simulink library "carnot"  (R2018b)
settings: Solver=VariableStepAuto  StartTime=0.0  StopTime=10.0  RelTol=1e-3
undefined symbols (not defined in the file or in its folder): A, A_earth, acol, Acol, ActPower1, ActPower2, ActPower3, Ad, Ad0, Ar, Au, Au0, Azimuth_Angle, B, Bd, Bd0, Br, Bu, Bu0, C, c1, c2, c3, c33, c4, c5, c6, CarnotCallbacks_Density, CarnotCallbacks_Enthalpy, CarnotCallbacks_Enthalpy2Temperature, CarnotCallbacks_Entropy, CarnotCallbacks_Evaporation_Enthalpy, CarnotCallbacks_GlobalMessageLevel, CarnotCallbacks_Grashof, CarnotCallbacks_Heat_Capacity, CarnotCallbacks_Kinematic_Viscosity, CarnotCallbacks_PMV_PPD, CarnotCallbacks_Prandtl, CarnotCallbacks_Saturation_Property, CarnotCallbacks_Saturation_Temperature, CarnotCallbacks_Saturation_Value_Water, CarnotCallbacks_Specific_Volume, CarnotCallbacks_Thermal_Conductivity, CarnotCallbacks_Vapour_Content, CarnotCallbacks_Vapour_Pressure, Cd, Cdl, Cr, Cu, Davies, Dd, DE_TRY2010_04_averageYear, delta_grd, density, DiameterLastPiece, dl, DPConstant, DPLinear, DPQuadratic, Dr ... (+59)
libraries: $bdroot x429, simulink x36, simulink_extras x12
(part 14 of 22)

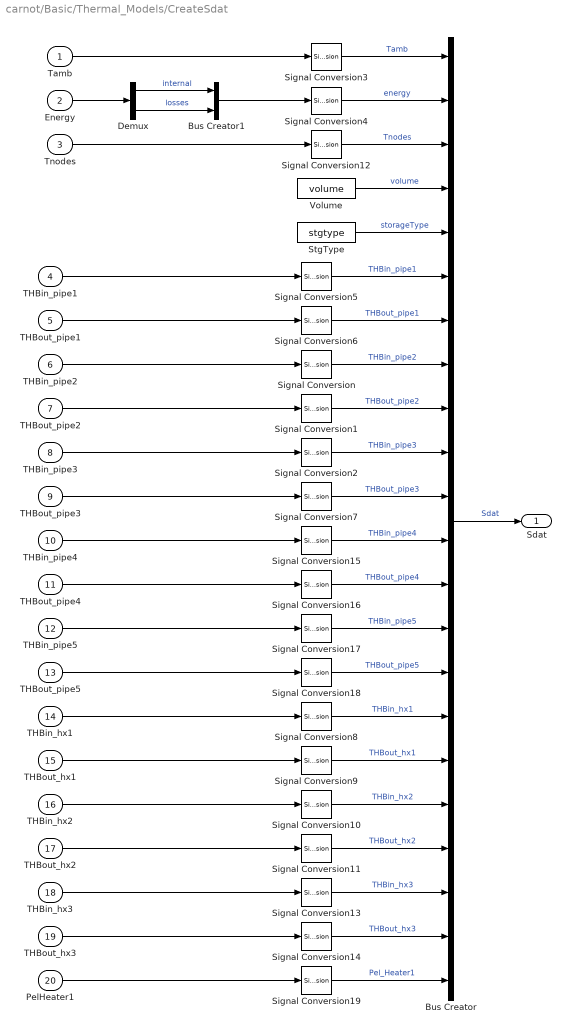
== system carnot/Basic/Thermal_Models/CreateSdat ==
  Tamb : Inport
  Energy : Inport  Port=2
  Tnodes : Inport  Port=3
  THBin_pipe1 : Inport  Port=4
  THBout_pipe1 : Inport  Port=5
  THBin_pipe2 : Inport  Port=6
  THBout_pipe2 : Inport  Port=7
  THBin_pipe3 : Inport  Port=8
  THBout_pipe3 : Inport  Port=9
  THBin_pipe4 : Inport  Port=10
  THBout_pipe4 : Inport  Port=11
  THBin_pipe5 : Inport  Port=12
  THBout_pipe5 : Inport  Port=13
  THBin_hx1 : Inport  Port=14
  THBout_hx1 : Inport  Port=15
  THBin_hx2 : Inport  Port=16
  THBout_hx2 : Inport  Port=17
  THBin_hx3 : Inport  Port=18
  THBout_hx3 : Inport  Port=19
  PelHeater1 : Inport  Port=20
  Bus Creator : BusCreator  Inputs=22
  Bus Creator1 : BusCreator  Inputs=2
  Demux : Demux  Outputs=2
  Signal Conversion{,1..19} (20 alike) : SignalConversion  OverrideOpt=off
  StgType : Constant  Value=stgtype
  Volume : Constant  Value=volume
  Sdat : Outport
  wires:
  Volume/1 -> Bus Creator/4  "volume"
  Bus Creator1/1 -> Signal Conversion4/1
  Energy/1 -> Demux/1
  Demux/1 -> Bus Creator1/1  "internal"
  Demux/2 -> Bus Creator1/2  "losses"
  Signal Conversion3/1 -> Bus Creator/1  "Tamb"
  THBin_pipe2/1 -> Signal Conversion/1
  Signal Conversion5/1 -> Bus Creator/6  "THBin_pipe1"
  Signal Conversion7/1 -> Bus Creator/11  "THBout_pipe3"
  THBout_pipe3/1 -> Signal Conversion7/1
  Signal Conversion10/1 -> Bus Creator/18  "THBin_hx2"
  Tnodes/1 -> Signal Conversion12/1
  THBin_pipe3/1 -> Signal Conversion2/1
  Tamb/1 -> Signal Conversion3/1
  Signal Conversion8/1 -> Bus Creator/16  "THBin_hx1"
  Signal Conversion4/1 -> Bus Creator/2  "energy"
  Signal Conversion9/1 -> Bus Creator/17  "THBout_hx1"
  THBout_pipe2/1 -> Signal Conversion1/1
  Signal Conversion6/1 -> Bus Creator/7  "THBout_pipe1"
  Signal Conversion12/1 -> Bus Creator/3  "Tnodes"
  THBin_hx1/1 -> Signal Conversion8/1
  THBout_hx1/1 -> Signal Conversion9/1
  THBin_hx2/1 -> Signal Conversion10/1
  Bus Creator/1 -> Sdat/1  "Sdat"
  THBin_pipe1/1 -> Signal Conversion5/1
  THBout_hx2/1 -> Signal Conversion11/1
  THBout_pipe1/1 -> Signal Conversion6/1
  Signal Conversion1/1 -> Bus Creator/9  "THBout_pipe2"
  Signal Conversion/1 -> Bus Creator/8  "THBin_pipe2"
  Signal Conversion2/1 -> Bus Creator/10  "THBin_pipe3"
  Signal Conversion11/1 -> Bus Creator/19  "THBout_hx2"
  Signal Conversion13/1 -> Bus Creator/20  "THBin_hx3"
  THBin_hx3/1 -> Signal Conversion13/1
  THBout_hx3/1 -> Signal Conversion14/1
  Signal Conversion14/1 -> Bus Creator/21  "THBout_hx3"
  StgType/1 -> Bus Creator/5  "storageType"
  Signal Conversion15/1 -> Bus Creator/12  "THBin_pipe4"
  THBin_pipe4/1 -> Signal Conversion15/1
  THBout_pipe4/1 -> Signal Conversion16/1
  Signal Conversion16/1 -> Bus Creator/13  "THBout_pipe4"
  Signal Conversion18/1 -> Bus Creator/15  "THBout_pipe5"
  THBout_pipe5/1 -> Signal Conversion18/1
  THBin_pipe5/1 -> Signal Conversion17/1
  Signal Conversion17/1 -> Bus Creator/14  "THBin_pipe5"
  PelHeater1/1 -> Signal Conversion19/1
  Signal Conversion19/1 -> Bus Creator/22  "Pel_Heater1"

== system carnot/Basic/Thermal_Models/Floor_in ==
  "[AIV]floor" : Inport
  power per node : Inport  Port=2
  "[AIV]ceiling" : Inport  Port=3
  Qdot_sol : Inport  Port=4
  Mux : Mux  Inputs=3
  Wall_basic : $bdroot/Basic/Thermal_Models/Wall_basic  tau=tau  t0=t0  d=d  dactive=dactive  cond=cond  cwall=cwall  rho=rho
  alfa_ceiling : $bdroot/Basic/Heat_Transfer/alfa_ceiling  active=active  emission_c=emission_c  wallsurface=wallsurface
  alfa_floor : $bdroot/Basic/Heat_Transfer/alfa_floor  active=active  emission_f=emission_f  wallsurface=wallsurface
  per surface : Gain  Gain=1/wallsurface  SaturateOnIntegerOverflow=on  OutDataTypeStr=Inherit: Same as input  ParamDataTypeStr=Inherit: Same as input
  "[S]floor" : Outport
  T(P) : Outport  Port=2
  "[S]ceiling" : Outport  Port=3
  Tn : Outport  Port=4
  wires:
  Wall_basic/2 -> Mux/2, T(P)/1
  "[AIV]ceiling"/1 -> alfa_ceiling/2
  alfa_ceiling/2 -> "[S]ceiling"/1
  alfa_floor/2 -> "[S]floor"/1
  "[AIV]floor"/1 -> alfa_floor/2
  Wall_basic/3 -> Mux/3, alfa_ceiling/1
  Wall_basic/1 -> Mux/1, alfa_floor/1
  alfa_floor/1 -> Wall_basic/1
  alfa_ceiling/1 -> Wall_basic/3
  Qdot_sol/1 -> alfa_floor/3
  power per node/1 -> per surface/1
  per surface/1 -> Wall_basic/2
  Mux/1 -> Tn/1

== system carnot/Basic/Thermal_Models/HeatPump_basic ==
  THBin_source : Inport
  THBin_load : Inport  Port=2
  Tamb : Inport  Port=3
  Ctrl : Inport  Port=4
  Bus Assignment : BusAssignment  AssignedSignals=Temperature
  Bus Assignment1 : BusAssignment  AssignedSignals=Temperature
  Bus Creator : BusCreator  Inputs=7
  Bus Selector : BusSelector  OutputSignals=Temperature,MassFlow,Pressure,FluidType,FluidMix
  Bus Selector1 : BusSelector  OutputSignals=Temperature,MassFlow,Pressure,FluidType,FluidMix
  P_el calculus : Subsystem
  Product : DotProduct  InputSameDT=on  OutDataTypeStr=Inherit: Inherit via internal rule
  Product1 : DotProduct  InputSameDT=on  OutDataTypeStr=Inherit: Inherit via internal rule
  Product3 : DotProduct  InputSameDT=on  OutDataTypeStr=Inherit: Inherit via internal rule
  Sum1 : Sum  Inputs=+-  SaturateOnIntegerOverflow=on  InputSameDT=on  OutDataTypeStr=Inherit: Same as first input
  Sum2 : Sum  Inputs=+-  SaturateOnIntegerOverflow=on  InputSameDT=on  OutDataTypeStr=Inherit: Same as first input
  model cold side : Subsystem
  model hot side : Subsystem
  THBsource : Outport
  THBload : Outport  Port=2
  HPdat : Outport  Port=3
  wires:
  Product/1 -> Bus Creator/6  "Qdot_hot"
  Product3/1 -> Bus Creator/3  "Qdot_cold"
  model cold side/2(mdot*cp) -> Product3/2
  Sum1/1 -> Product3/1
  Bus Selector1/2 -> model cold side/2(mdot_cold)  "<MassFlow>"
  Ctrl/1 -> model hot side/8(command), Product1/1, model cold side/8(command)
  model hot side/2(Thot_out) -> Sum2/1, P_el calculus/1(Thot_out), model cold side/6(Thot), Bus Assignment/2
  Product1/1 -> Bus Creator/7  "Pelec"
  P_el calculus/1(P_el) -> Product1/2
  Bus Selector/3 -> model hot side/4(p_hot)  "<Pressure>"
  model cold side/1(Tcold_out) -> Bus Assignment1/2, Sum1/2
  Bus Selector1/1 -> model cold side/1(Tcold), Sum1/1, model hot side/1(Tcold), P_el calculus/2(Tcold_in)  "<Temperature>"
  Sum2/1 -> Product/2
  model hot side/1(mdot*cp) -> Product/1
  Bus Selector/2 -> model hot side/3(mdot_hot)  "<MassFlow>"
  Bus Selector/1 -> model hot side/2(Thot), Sum2/2  "<Temperature>"
  Bus Selector/5 -> model hot side/6(mix_hot)  "<FluidMix>"
  Bus Selector/4 -> model hot side/5(fluid_hot)  "<FluidType>"
  Bus Selector1/3 -> model cold side/3(p_cold)  "<Pressure>"
  Bus Selector1/4 -> model cold side/4(fluid_cold)  "<FluidType>"
  Bus Selector1/5 -> model cold side/5(mix_cold)  "<FluidMix>"
  THBin_load/1 -> Bus Selector/1, Bus Assignment/1, Bus Creator/4  "THBin_hot"
  Tamb/1 -> model cold side/7(Tamb), model hot side/7(Tamb)
  Bus Assignment/1 -> THBload/1, Bus Creator/5  "THBout_hot"
  THBin_source/1 -> Bus Selector1/1, Bus Assignment1/1, Bus Creator/1  "THBin_cold"
  Bus Assignment1/1 -> THBsource/1, Bus Creator/2  "THBout_cold"
  Bus Creator/1 -> HPdat/1

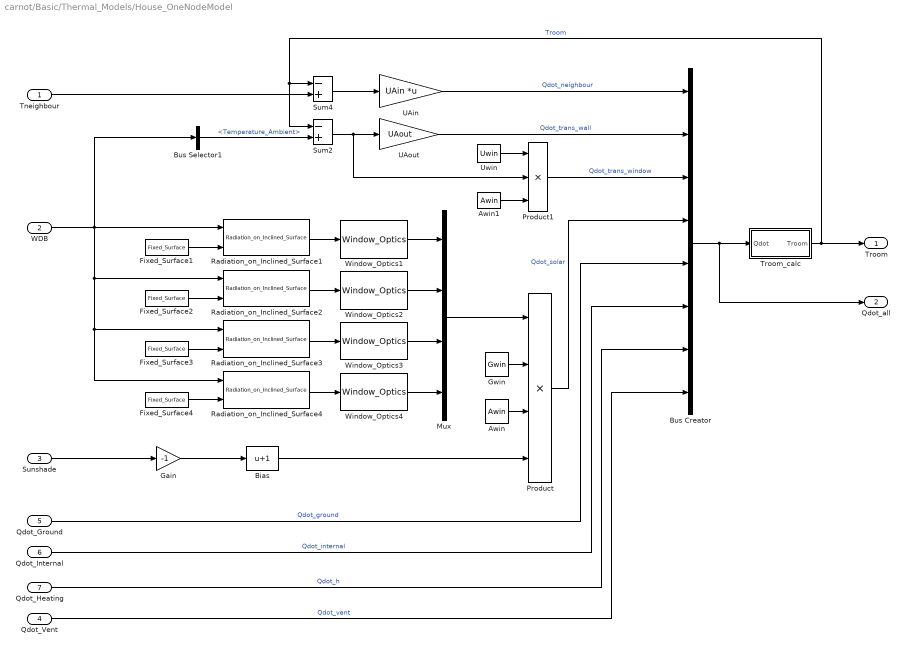
== system carnot/Basic/Thermal_Models/House_OneNodeModel ==
  Tneighbour : Inport
  WDB : Inport  Port=2
  Sunshade : Inport  Port=3
  Qdot_Vent : Inport  Port=4
  Qdot_Ground : Inport  Port=5
  Qdot_Internal : Inport  Port=6
  Qdot_Heating : Inport  Port=7
  Awin : Constant  Value=Awin
  Awin1 : Constant  Value=Awin
  Bias : Bias  Bias=1
  Bus Creator : BusCreator  Inputs=8
  Bus Selector1 : BusSelector  OutputSignals=Temperature_Ambient
  Fixed_Surface1 : $bdroot/Weather/Fixed_Surface  colangle=90  colazi=AziWin(1)  colrot=0
  Fixed_Surface2 : $bdroot/Weather/Fixed_Surface  colangle=90  colazi=AziWin(2)  colrot=0
  Fixed_Surface3 : $bdroot/Weather/Fixed_Surface  colangle=90  colazi=AziWin(3)  colrot=0
  Fixed_Surface4 : $bdroot/Weather/Fixed_Surface  colangle=90  colazi=AziWin(4)  colrot=0
  Gain : Gain  Gain=-1
  Gwin : Constant  Value=Gwin
  Mux : Mux
  Product : Product  Inputs=4
  Product1 : Product  Inputs=3
  Radiation_on_Inclined_Surface{1..4} (4 alike) : $bdroot/Weather/Radiation_on_Inclined_Surface  sky=Perez 1990  reflect=0.2
  Sum2 : Sum  Inputs=-+  SaturateOnIntegerOverflow=on  InputSameDT=on  OutDataTypeStr=Inherit: Same as first input
  Sum4 : Sum  Inputs=-+  SaturateOnIntegerOverflow=on  InputSameDT=on  OutDataTypeStr=Inherit: Same as first input
  Troom_calc : Subsystem  mask(Calculate room temperature){A=A, capa=capa, tini=tini, dtroom=dtroom}
      mask prompts: A "Heated surface of the house in m²"; capa "Thermal capactiy per surface in J/m²/K"; tini "Initial temperature in °C"; dtroom "Max. change of room temperature in K"
      mask help:
      | One node thermal model based on energy balance.
      | The room temperature can be limited by "Max. change of room temperature" . The temperature is limited by this parameter, the result of the energy balance (Qdot_all) is the required power to maintain the limit.
      mask TypeOptions A: A/Value
      mask TypeOptions capa: capa/Value
      mask TypeOptions tini: Tini/Value | add_Tini/Bias
  UAin : Gain  Gain=UAin  Multiplication=Matrix(K*u)  SaturateOnIntegerOverflow=on  OutDataTypeStr=Inherit: Same as input  ParamDataTypeStr=Inherit: Same as input
  UAout : Gain  Gain=UAout  SaturateOnIntegerOverflow=on  OutDataTypeStr=Inherit: Same as input  ParamDataTypeStr=Inherit: Same as input
  Uwin : Constant  Value=Uwin
  Window_Optics{1..4} (4 alike) : $bdroot/Basic/Thermal_Models/Window_Optics  BreakpointsForDimension1=[-10 0 50 70 80 90]  Table="[1.0 1.0  0.95  0.7  0.0  0.0]"  Gain=0.8
  Troom : Outport
  Qdot_all : Outport  Port=2
  wires:
  Bias/1 -> Product/4
  Gain/1 -> Bias/1
  Uwin/1 -> Product1/1
  Awin1/1 -> Product1/3
  Awin/1 -> Product/3
  Gwin/1 -> Product/2
  Tneighbour/1 -> Sum4/2
  Qdot_Vent/1 -> Bus Creator/8  "Qdot_vent"
  Sunshade/1 -> Gain/1
  Mux/1 -> Product/1
  Qdot_Heating/1 -> Bus Creator/7  "Qdot_h"
  Window_Optics4/1 -> Mux/4
  Window_Optics3/1 -> Mux/3
  Window_Optics2/1 -> Mux/2
  Window_Optics1/1 -> Mux/1
  Product/1 -> Bus Creator/4  "Qdot_solar"
  Sum2/1 -> UAout/1, Product1/2
  UAout/1 -> Bus Creator/2  "Qdot_trans_wall"
  Bus Selector1/1 -> Sum2/2  "<Temperature_Ambient>"
  WDB/1 -> Bus Selector1/1, Radiation_on_Inclined_Surface4/1, Radiation_on_Inclined_Surface3/1, Radiation_on_Inclined_Surface2/1, Radiation_on_Inclined_Surface1/1
  Bus Creator/1 -> Qdot_all/1, Troom_calc/1(Qdot)
  Qdot_Ground/1 -> Bus Creator/5  "Qdot_ground"
  Sum4/1 -> UAin/1
  UAin/1 -> Bus Creator/1  "Qdot_neighbour"
  Fixed_Surface1/1 -> Radiation_on_Inclined_Surface1/2
  Radiation_on_Inclined_Surface1/1 -> Window_Optics1/1
  Fixed_Surface2/1 -> Radiation_on_Inclined_Surface2/2
  Radiation_on_Inclined_Surface2/1 -> Window_Optics2/1
  Fixed_Surface3/1 -> Radiation_on_Inclined_Surface3/2
  Radiation_on_Inclined_Surface3/1 -> Window_Optics3/1
  Fixed_Surface4/1 -> Radiation_on_Inclined_Surface4/2
  Radiation_on_Inclined_Surface4/1 -> Window_Optics4/1
  Troom_calc/1(Troom) -> Troom/1, Sum4/1, Sum2/1  "Troom"
  Product1/1 -> Bus Creator/3  "Qdot_trans_window"
  Qdot_Internal/1 -> Bus Creator/6  "Qdot_internal"

== system carnot/Basic/Thermal_Models/Pipe_basic ==
  Tamb : Inport
  THBin : Inport  Port=2
  Bus Assignment : BusAssignment  AssignedSignals=Temperature
  Bus Selector : BusSelector  OutputSignals=Temperature,MassFlow,Pressure,FluidType,FluidMix
  S-Function : S-Function  FunctionName=pipe_Tnodes  Parameters="vnode, lnode,  unode,  cond,  cnode,  t0, nodes"  SFunctionDeploymentMode=off  EnableBusSupport=off
  Tnodes : Outport
  THB : Outport  Port=2
  wires:
  THBin/1 -> Bus Assignment/1, Bus Selector/1
  S-Function/1 -> Bus Assignment/2
  Tamb/1 -> S-Function/1
  Bus Selector/1 -> S-Function/2  "<Temperature>"
  Bus Selector/2 -> S-Function/3  "<MassFlow>"
  Bus Selector/3 -> S-Function/4  "<Pressure>"
  Bus Selector/4 -> S-Function/5  "<FluidType>"
  Bus Selector/5 -> S-Function/6  "<FluidMix>"
  S-Function/2 -> Tnodes/1
  Bus Assignment/1 -> THB/1

== system carnot/Basic/Thermal_Models/Radiator_basic ==
  note: One node model with upwind scheme. Power balance is:
      | m*cp*dTnode/dt = -qdot + mdot*cp*(Tin - Tnode)
      |
      | EN 442:
      | qdot = qdot_nominal * ((Tnode-Troom)/(Tdiff_nominal)^expo
      | nominal temperature difference = 50K with flowline 75°C, return 65°C and room 20°C
      | in EN, the Tnode is mean temperature Tm = 0.5*(Tin+Tout)
      |
      | Here Tout = Tnode in difference to EN442
      | A correction of expo and nominal power is done in the mask.
  THB_in : Inport
  Troom : Inport  Port=2
  Abs : Abs  SaturateOnIntegerOverflow=on
  Bus Selector : BusSelector  OutputSignals=Temperature,MassFlow
  Gain : Gain  Gain=1/dtnom  SaturateOnIntegerOverflow=on  OutDataTypeStr=Inherit: Same as input  ParamDataTypeStr=Inherit: Same as input
  Gain1 : Gain  Gain=pnom  SaturateOnIntegerOverflow=on  OutDataTypeStr=Inherit: Same as input  ParamDataTypeStr=Inherit: Same as input
  Heat_Capacity : $bdroot/Basic/Material_Properties/Heat_Capacity  VariantControl=CarlibClassic  INPUTARGUMENTS=THB  DEBUGLEVEL=DEBUGLEVEL  MAXTOTALWARNINGS=inf  MAXCONSECUTIVEWARNINGS=inf  WRITETOFILE=0  FILENAME='errors.txt'
  Math Function : Math  Operator=pow  SaturateOnIntegerOverflow=on
  Product : Product  Inputs=3  SaturateOnIntegerOverflow=on  InputSameDT=on  OutDataTypeStr=Inherit: Same as first input
  Product1 : Product  SaturateOnIntegerOverflow=on  InputSameDT=on  OutDataTypeStr=Inherit: Same as first input
  Sign : Signum
  Sum : Sum  Inputs=-+  SaturateOnIntegerOverflow=on  InputSameDT=on  OutDataTypeStr=Inherit: Same as first input
  Sum1 : Sum  Inputs=-+  SaturateOnIntegerOverflow=on  InputSameDT=on  OutDataTypeStr=Inherit: Same as first input
  Sum3 : Sum  Inputs=-+  SaturateOnIntegerOverflow=on  InputSameDT=on  OutDataTypeStr=Inherit: Same as first input
  THB_set_T : $bdroot/Source/Simple/THB_set_T
  Transfer Fcn (with initial states) : simulink_extras/Additional Linear/Transfer Fcn (with initial states)  N=[1]  D="[mcap  0]"  X0=tini*mcap
  const : Constant  Value=expo
  THB : Outport
  Qdot2room : Outport  Port=2
  wires:
  Troom/1 -> Sum3/1
  Bus Selector/1 -> Sum/2  "<Temperature>"
  Sign/1 -> Product1/2
  Sum3/1 -> Sign/1, Gain/1
  Gain1/1 -> Product1/1
  Abs/1 -> Math Function/1
  Gain/1 -> Abs/1
  Math Function/1 -> Gain1/1
  const/1 -> Math Function/2
  Product1/1 -> Qdot2room/1, Sum1/1
  Sum/1 -> Product/1
  Bus Selector/2 -> Product/2  "<MassFlow>"
  Heat_Capacity/1 -> Product/3
  Product/1 -> Sum1/2
  Sum1/1 -> Transfer Fcn (with initial states)/1
  Transfer Fcn (with initial states)/1 -> Sum3/2, Sum/1, THB_set_T/2
  THB_set_T/1 -> THB/1
  THB_in/1 -> Bus Selector/1, Heat_Capacity/1, THB_set_T/1

== system carnot/Basic/Thermal_Models/Roof ==
  WDB : Inport
  power per node : Inport  Port=2
  "[AIV]" : Inport  Port=3
  Mux : Mux  Inputs=3
  Wall_basic : $bdroot/Basic/Thermal_Models/Wall_basic  tau=tau  t0=t0  d=d  dactive=dactive  cond=cond  cwall=cwall  rho=rho
  alfa_ceiling : $bdroot/Basic/Heat_Transfer/alfa_ceiling  active=active  emission_c=emission_c  wallsurface=wallsurface
  alfa_wall_out : $bdroot/Basic/Heat_Transfer/alfa_wall_out  pos=pos  absorption_out=absorption_out  emission_out=emission_out  wallsurface=wallsurface
  per surface : Gain  Gain=1/wallsurface  SaturateOnIntegerOverflow=on  OutDataTypeStr=Inherit: Same as input  ParamDataTypeStr=Inherit: Same as input
  "[S]" : Outport
  Tn : Outport  Port=2
  wires:
  per surface/1 -> Wall_basic/2
  power per node/1 -> per surface/1
  alfa_ceiling/2 -> "[S]"/1
  "[AIV]"/1 -> alfa_ceiling/2
  alfa_ceiling/1 -> Wall_basic/3
  Wall_basic/2 -> Mux/2
  Wall_basic/3 -> Mux/3, alfa_ceiling/1
  Wall_basic/1 -> Mux/1, alfa_wall_out/2
  WDB/1 -> alfa_wall_out/1
  alfa_wall_out/1 -> Wall_basic/1
  Mux/1 -> Tn/1

== system carnot/Basic/Thermal_Models/Room_Node ==
  note: NODE of a ZONE ( heat flow, temperature, ventilation / infiltration and energy consumption)
  note: r: radiative
      | c: convective
  sum([S]) : Inport
  1/s to 1/h : Gain  Gain=3600  SaturateOnIntegerOverflow=on  OutDataTypeStr=Inherit: Same as input  ParamDataTypeStr=Inherit: Same as input
  Demux2 : Demux  Outputs=13
  Mux2 : Mux  Inputs=6
  Mux3 : Mux  Inputs=9
  Sensitive room temperature : Subsystem  mask(SENSITIVE TEMPERATURE){share_c=47}
      mask prompts: share_c "SHARE of convective sensitivity, [0,100%]:"
      mask help:
      | This block merges the convective and radiative zone node temperature to the SENSITIVE ZONE TEMPERATURE (weighted arithmetic average of both components).
      |
      | [T] = [Tc; Tr]:  temperature vector of node, °C
      | Ts:              sensitive zone temperature, °C
      mask init: same as carnot/Outputs/Sensitive_Room_Temperature
  Terminator : Terminator
  convective_node : Subsystem
  m^3 : Constant  Value=zoneairvolume
  radiative_node : Subsystem
  "[AIV]" : Outport
  "[S]" : Outport  Port=2
  Qdot_sol : Outport  Port=3
  Vair : Outport  Port=4
  wires:
  Sensitive room temperature/1(Ts) -> Mux3/1  "Ts"
  Mux3/1 -> "[AIV]"/1
  Demux2/13 -> convective_node/6(Vdot_in2out)  "Vdot_in2out"
  Demux2/12 -> convective_node/5(Vdot_out2in)  "Vdot_out2in"
  Demux2/11 -> convective_node/4(D_mdot_CO2)  "delta_mdot_CO2"
  Demux2/10 -> convective_node/3(D_mdot_H2O)  "delta_mdot_H2O"
  Demux2/9 -> convective_node/2(D_mdot_air)  "delta_mdot_air"
  radiative_node/1(Tr) -> Mux3/3, Sensitive room temperature/1(Tr)  "Tr"
  convective_node/1(Tc) -> Mux3/2, Sensitive room temperature/2(Tc)  "Tc"
  convective_node/7(nair_out) -> 1/s to 1/h/1
  convective_node/4(rho) -> Mux3/6  "rho"
  convective_node/5(cp) -> Mux3/7  "cp"
  convective_node/6(p) -> Mux3/8  "p"
  convective_node/3(x_CO2) -> Mux3/5  "x_CO2"
  convective_node/2(x_H2O) -> Mux3/4  "x_H2O"
  1/s to 1/h/1 -> Mux3/9  "nair_out"
  Demux2/1 -> Qdot_sol/1, Mux2/1  "Qdot_sol"
  Demux2/2 -> Mux2/2  "Qdot_equip"
  Demux2/3 -> Mux2/3  "Qdot_light"
  Demux2/4 -> Mux2/4  "Qdot_pers"
  Demux2/5 -> Mux2/5  "Qdot_heat"
  Demux2/6 -> Mux2/6  "Qdot_air"
  Demux2/7 -> convective_node/1(Qdotc)  "Qdotc"
  Demux2/8 -> radiative_node/1(Qdotr)  "Qdotr"
  sum([S])/1 -> Demux2/1, "[S]"/1
  Mux2/1 -> Terminator/1  "[Qdot]"
  m^3/1 -> Vair/1

== system carnot/Basic/Thermal_Models/Solar_Collector_basic ==
  solar : Inport
  THB : Inport  Port=2
  Bus Selector1 : BusSelector  OutputSignals=Temperature,MassFlow
  Bus Selector2 : BusSelector  OutputSignals=Pressure,FluidType,FluidMix  OutputAsBus=on
  S-Function : S-Function  FunctionName=solarcollector12975  Parameters=acol, c1, c2, c3, c4, c5, c6, tini  SFunctionDeploymentMode=off  EnableBusSupport=off
  Tout : Outport
  Tmean : Outport  Port=2
  Qdot : Outport  Port=3
  wires:
  Bus Selector1/2 -> S-Function/3  "<MassFlow>"
  Bus Selector1/1 -> S-Function/2  "<Temperature>"
  Bus Selector2/1 -> S-Function/4
  THB/1 -> Bus Selector1/1, Bus Selector2/1
  solar/1 -> S-Function/1
  S-Function/1 -> Tout/1  "Tout"
  S-Function/2 -> Tmean/1  "Tmean"
  S-Function/3 -> Qdot/1  "power"

== system carnot/Basic/Thermal_Models/T_Ground_Undisturbed ==
  note: u(1) - u(2)*exp(-u(3)/u(4))*cos(2*pi*(u(5)-u(6)*3600)/(365*24*3600) - u(3)/u(4)) + 0.03*u(3)
  -1/delta_grd : Gain  Gain=-1/delta_grd
  Math Function : Math  SaturateOnIntegerOverflow=on
  Product : Product  RndMeth=Zero
  Sine Wave : Sin  Amplitude=deltathetae  Frequency=2*pi/(365*24*3600)  Phase=pi/2 - 2*pi*tshift/(365*24) - z/delta_grd  SampleTime=0
  Sum : Sum  Inputs=+-+
  Tmeanoutside1 : Constant  Value=Tmeanoutside
  gain : Gain  Gain=0.03
  height vector : Constant  Value=z
  Tearth : Outport
  wires:
  Tmeanoutside1/1 -> Sum/1
  Sum/1 -> Tearth/1
  Product/1 -> Sum/2
  Sine Wave/1 -> Product/2
  Math Function/1 -> Product/1
  -1/delta_grd/1 -> Math Function/1
  height vector/1 -> -1/delta_grd/1, gain/1
  gain/1 -> Sum/3

== system carnot/Basic/Thermal_Models/ThermalNodeTHB ==
  THB : Inport
  Bus Selector : BusSelector  OutputSignals=Temperature,MassFlow
  Const : Constant  Value=0
  Heat_Capacity : $bdroot/Basic/Material_Properties/Heat_Capacity  VariantControl=CarlibClassic  INPUTARGUMENTS=THB  DEBUGLEVEL=DEBUGLEVEL  MAXTOTALWARNINGS=inf  MAXCONSECUTIVEWARNINGS=inf  WRITETOFILE=0  FILENAME='errors.txt'
  Tamb : Constant  Value=Tini
  Thermal_Node : $bdroot/Basic/Thermal_Models/Thermal_Node  UA=UA  mcp=mcp
  T : Outport  InitialOutput=20
  wires:
  Tamb/1 -> Thermal_Node/1
  Heat_Capacity/1 -> Thermal_Node/5
  THB/1 -> Heat_Capacity/1, Bus Selector/1
  Bus Selector/2 -> Thermal_Node/3  "<MassFlow>"
  Bus Selector/1 -> Thermal_Node/2  "<Temperature>"
  Thermal_Node/1 -> T/1
  Const/1 -> Thermal_Node/4

== system carnot/Basic/Thermal_Models/Thermal_Node ==
  Tamb : Inport
  Tin : Inport  Port=2
  mdot : Inport  Port=3
  Qdot : Inport  Port=4
  cp : Inport  Port=5
  Divide : Product  Inputs=*/
  Integrator : Integrator  InitialConditionSource=external  InitialCondition=40
  Losses : Gain  Gain=UA  SaturateOnIntegerOverflow=on  OutDataTypeStr=Inherit: Same as input  ParamDataTypeStr=Inherit: Same as input
  Mux : Mux  Inputs=3
  Product1 : Product  Inputs=3  SaturateOnIntegerOverflow=on  InputSameDT=on  OutDataTypeStr=Inherit: Same as first input
  Sum1 : Sum  Inputs=-+  SaturateOnIntegerOverflow=on  InputSameDT=on  OutDataTypeStr=Inherit: Same as first input
  Sum3 : Sum  Inputs=-+  SaturateOnIntegerOverflow=on  InputSameDT=on  OutDataTypeStr=Inherit: Same as first input
  Sum4 : Sum  Inputs=1  SaturateOnIntegerOverflow=on  InputSameDT=on  OutDataTypeStr=Inherit: Same as first input
  nodeCapacity : Constant  Value=mcp
  Tout : Outport  InitialOutput=40
  wires:
  Sum4/1 -> Divide/1
  nodeCapacity/1 -> Divide/2
  mdot/1 -> Product1/2
  Tin/1 -> Sum1/2
  Integrator/1 -> Tout/1, Sum1/1, Sum3/1  "Tout"
  Product1/1 -> Mux/2
  Mux/1 -> Sum4/1
  Tamb/1 -> Sum3/2, Integrator/2
  Losses/1 -> Mux/1
  Sum3/1 -> Losses/1
  cp/1 -> Product1/3
  Divide/1 -> Integrator/1
  Sum1/1 -> Product1/1
  Qdot/1 -> Mux/3

== system carnot/Basic/Thermal_Models/Wall_basic ==
  qdot_in : Inport
  QdotActive : Inport  Port=2
  qdot_out : Inport  Port=3
  S-Function : S-Function  FunctionName=layerwall  Parameters=tau, t0, d, cond, cwall, rho, dactive  SFunctionDeploymentMode=off  EnableBusSupport=off
  Tin : Outport
  Tactive : Outport  Port=2
  Tout : Outport  Port=3
  wires:
  qdot_in/1 -> S-Function/1
  S-Function/1 -> Tin/1
  QdotActive/1 -> S-Function/2
  S-Function/2 -> Tactive/1  "T(active)"
  qdot_out/1 -> S-Function/3
  S-Function/3 -> Tout/1

== system carnot/Basic/Thermal_Models/Wall_in ==
  "[AIV]" : Inport
  power per node : Inport  Port=2
  "[AIV]n" : Inport  Port=3
  Mux : Mux  Inputs=3
  Wall_basic : $bdroot/Basic/Thermal_Models/Wall_basic  tau=tau  t0=t0  d=d  dactive=dactive  cond=cond  cwall=cwall  rho=rho
  alfa_wall_in : $bdroot/Basic/Heat_Transfer/alfa_wall_in  active=active  emission_in=emission_in  wallsurface=wallsurface
  alfa_wall_in1 : $bdroot/Basic/Heat_Transfer/alfa_wall_in  active=active  emission_in=emission_in  wallsurface=wallsurface
  per surface : Gain  Gain=1/wallsurface  SaturateOnIntegerOverflow=on  OutDataTypeStr=Inherit: Same as input  ParamDataTypeStr=Inherit: Same as input
  "[S]" : Outport
  "[S]n" : Outport  Port=2
  Tn : Outport  Port=3
  wires:
  Mux/1 -> Tn/1
  Wall_basic/2 -> Mux/2
  alfa_wall_in1/2 -> "[S]n"/1
  "[AIV]n"/1 -> alfa_wall_in1/2
  Wall_basic/3 -> alfa_wall_in1/1, Mux/3
  alfa_wall_in1/1 -> Wall_basic/3
  "[AIV]"/1 -> alfa_wall_in/2
  Wall_basic/1 -> Mux/1, alfa_wall_in/1
  alfa_wall_in/2 -> "[S]"/1
  alfa_wall_in/1 -> Wall_basic/1
  per surface/1 -> Wall_basic/2
  power per node/1 -> per surface/1

== system carnot/Basic/Thermal_Models/Wall_out ==
  WDB : Inport
  power per node : Inport  Port=2
  "[AIV]" : Inport  Port=3
  Mux : Mux  Inputs=3
  Wall_basic : $bdroot/Basic/Thermal_Models/Wall_basic  tau=tau  t0=t0  d=d  dactive=dactive  cond=cond  cwall=cwall  rho=rho
  alfa_wall_in : $bdroot/Basic/Heat_Transfer/alfa_wall_in  active=active  emission_in=emission_in  wallsurface=wallsurface
  alfa_wall_out : $bdroot/Basic/Heat_Transfer/alfa_wall_out  pos=pos  absorption_out=absorption_out  emission_out=emission_out  wallsurface=wallsurface
  per surface : Gain  Gain=1/wallsurface  SaturateOnIntegerOverflow=on  OutDataTypeStr=Inherit: Same as input  ParamDataTypeStr=Inherit: Same as input
  "[S]" : Outport
  Tn : Outport  Port=2
  wires:
  alfa_wall_in/2 -> "[S]"/1
  "[AIV]"/1 -> alfa_wall_in/2
  Wall_basic/3 -> Mux/3, alfa_wall_in/1
  alfa_wall_in/1 -> Wall_basic/3
  Wall_basic/1 -> Mux/1, alfa_wall_out/2
  alfa_wall_out/1 -> Wall_basic/1
  per surface/1 -> Wall_basic/2
  power per node/1 -> per surface/1
  WDB/1 -> alfa_wall_out/1
  Wall_basic/2 -> Mux/2
  Mux/1 -> Tn/1

== system carnot/Basic/Thermal_Models/Wall_with_Window ==
  WDB : Inport
  "[AIV]" : Inport  Port=2
  Ground : Ground
  Ground1 : Ground
  Wall_out : $bdroot/Basic/Thermal_Models/Wall_out  wallsize=[wallsize(1), wallsize(2)-windowsize(1)*windowsize(2)/wallsize(1)]  pos=pos  t0=t0  d=[0.1 0.38]  cond=[0.04 0.79]  cwall=[0.28 0.28]*3600  rho=[900 1800]  reflectground=0.3  abs_emiss=[0.65 0.97 0.96]  tau=tau  dactive=-1
  Window : $bdroot/Basic/Thermal_Models/Window  pos=pos  windowsize=windowsize  frame=frame  Ug=1.8  gvalue=g  tauzero=g*0.95  numpanes=2  d=[0.004 0.004]  rho=[2500 2500]  cp="[1008  1008]"  t0=t0  misc=[0.2 0.1 1 1]  shad_type=No shading  type_glazing=double glazing normal  tau_shad=0.01  bli_a=0.05  bli_b=1  bli_c=0.05  bli_d=0.05  bli_alpha=90  bli_refl=0.2
  "[S]wall" : Outport
  "[S]window" : Outport  Port=2
  TnWall : Outport  Port=3
  wires:
  Ground1/1 -> Window/3
  Window/1 -> "[S]window"/1
  Wall_out/1 -> "[S]wall"/1
  Ground/1 -> Wall_out/2
  "[AIV]"/1 -> Window/2, Wall_out/3
  WDB/1 -> Wall_out/1, Window/1
  Wall_out/2 -> TnWall/1

== system carnot/Basic/Thermal_Models/Window ==
  WDB : Inport
  "[AIV]" : Inport  Port=2
  control : Inport  Port=3
  alfa_window_in : $bdroot/Basic/Heat_Transfer/alfa_window_in  type_glazing=double glazing normal  gvalue=gvalue  tauzero=tauzero  emission_in=misc(4)  wallsurface=windowsurface  frame=frame  numlayer=numpanes  shad_type=No shading  tau_shad=tau_shad  bli_a=bli_a  bli_b=bli_b  bli_c=bli_c  bli_d=bli_d  bli_alpha=bli_alpha  bli_refl=bli_refl
  alfa_window_out : $bdroot/Basic/Heat_Transfer/alfa_window_out  pos=pos  absorption_out=absorption_out  emission_out=emission_out  frame=frame
  lambda_window : Subsystem  mask(LAMBDA){}
      mask help:
      | Heat conduction through a transparent component (window).
      |
      | qdots1	: specific heat flow vertical on surface 1, W/m²
      | qdots2	: specific heat flow vertical on surface 2, W/m²
      | Ts1	: temperature of surface 1, °C
      | Ts2	: temperature of surface 2, °C
      |
      | NOTE CONVENTION for INPUT NUMBER:
      | "1"	  indoor surface of an outer window OR
      | 	  surface "a" of an inner window OR
      |  	  surface "f" of a glass floor
      |
      | "2"	  outdoor surface of a window OR
      | 	  surface "b" of an inner window OR
      |  	  surface "c" of a glass ceiling
  position1 : Constant
  "[S]" : Outport
  wires:
  lambda_window/2(Ts2) -> alfa_window_in/1
  lambda_window/1(Ts1) -> alfa_window_out/3
  WDB/1 -> alfa_window_in/4, alfa_window_out/1
  "[AIV]"/1 -> alfa_window_in/3
  alfa_window_in/1 -> lambda_window/2(qdots2)
  alfa_window_in/2 -> "[S]"/1
  alfa_window_out/2 -> lambda_window/1(qdots1)
  alfa_window_out/1 -> alfa_window_in/2
  control/1 -> alfa_window_in/5
  position1/1 -> alfa_window_out/2

== system carnot/Basic/Thermal_Models/Window_Optics ==
  WDB : Inport
  Bus Selector : BusSelector  OutputSignals=Incidence_Angle_sun,Solar_Radiation_direct_surface,Solar_Radiation_diffuse_surface
  IAM diffuse : Gain  Gain=Gain  SaturateOnIntegerOverflow=on  OutDataTypeStr=Inherit: Same as input  ParamDataTypeStr=Inherit: Same as input
  IAM window : Lookup_n-D  NumberOfTableDimensions=1  BreakpointsForDimension1=BreakpointsForDimension1  BeginIndexSearchUsingPreviousIndexResult=on  Table=Table  InternalRulePriority=Speed  RndMeth=Simplest  InputSameDT=on
  Product : Product
  Sum : Sum  SaturateOnIntegerOverflow=on  InputSameDT=on  OutDataTypeStr=Inherit: Same as first input
  qsolar : Outport
  wires:
  Bus Selector/3 -> IAM diffuse/1  "<Solar_Radiation_diffuse_surface>"
  IAM window/1 -> Product/1
  IAM diffuse/1 -> Sum/2
  Product/1 -> Sum/1
  Sum/1 -> qsolar/1
  Bus Selector/1 -> IAM window/1  "<Incidence_Angle_sun>"
  Bus Selector/2 -> Product/2  "<Solar_Radiation_direct_surface>"
  WDB/1 -> Bus Selector/1

== system carnot/Basic/Thermal_Models/sfun_storage_heatexchanger ==
  Tnodes : Inport
  THBin : Inport  Port=2
  Bus Selector : BusSelector  OutputSignals=Temperature,MassFlow,Pressure,FluidType,FluidMix
  Mux1 : Mux  Inputs=5
  storeHX : S-Function  FunctionName=storage_heatexchanger  Parameters=id, nodes, inlet, outlet, p1, p2, p3, p4, p5, p6, p7  SFunctionDeploymentMode=off  EnableBusSupport=off  SFcnStateName=DWORK_TS_OLD
      settings: SFcnIsStateOwnerBlock=on
  Qnodes : Outport
  Thx : Outport  Port=2
  wires:
  Mux1/1 -> storeHX/2
  Bus Selector/5 -> Mux1/5  "<FluidMix>"
  Bus Selector/4 -> Mux1/4  "<FluidType>"
  Bus Selector/3 -> Mux1/3  "<Pressure>"
  Bus Selector/2 -> Mux1/2  "<MassFlow>"
  Bus Selector/1 -> Mux1/1  "<Temperature>"
  Tnodes/1 -> storeHX/1
  storeHX/1 -> Qnodes/1
  THBin/1 -> Bus Selector/1
  storeHX/2 -> Thx/1

== system carnot/Basic/Weather_and_Sun/Cloudage ==
  Iglob : Inport
  S : Constant  Value=latitude
  S-Function : S-Function  FunctionName=metcloud_s  Parameters=skytype  SFunctionDeploymentMode=off  EnableBusSupport=off
  S1 : Constant  Value=longitude
  S2 : Constant  Value=longitude0
  mux5 : Mux
  cloudage : Outport
  wires:
  S1/1 -> mux5/3
  S/1 -> mux5/2
  mux5/1 -> S-Function/1
  S2/1 -> mux5/4
  S-Function/1 -> cloudage/1
  Iglob/1 -> mux5/1

== system carnot/Basic/Weather_and_Sun/Radiation_Divison ==
  Iglob : Inport
  S : Constant  Value=latitude
  S-Function : S-Function  FunctionName=metrad_s  SFunctionDeploymentMode=off  EnableBusSupport=off
  S1 : Constant  Value=longitude
  S2 : Constant  Value=longitude0
  Idir : Outport
  Idfu : Outport  Port=2
  SunAngle : Outport  Port=3
  Zenith : Outport  Port=4
  Azimuth : Outport  Port=5
  Clearness : Outport  Port=6
  wires:
  S2/1 -> S-Function/4
  S1/1 -> S-Function/3
  S/1 -> S-Function/2
  Iglob/1 -> S-Function/1
  S-Function/1 -> Idir/1
  S-Function/2 -> Idfu/1
  S-Function/3 -> SunAngle/1
  S-Function/4 -> Zenith/1
  S-Function/5 -> Azimuth/1
  S-Function/6 -> Clearness/1

== system carnot/Basic/Weather_and_Sun/Sky_Temperature ==
  Tamb : Inport
  hum : Inport  Port=2
  cloudage : Inport  Port=3
  S-Function : S-Function  FunctionName=metsky_s  Parameters=tskymodel  SFunctionDeploymentMode=off  EnableBusSupport=off
  mux6 : Mux  Inputs=3
  Tsky : Outport
  wires:
  S-Function/1 -> Tsky/1
  mux6/1 -> S-Function/1
  Tamb/1 -> mux6/1
  hum/1 -> mux6/2
  cloudage/1 -> mux6/3

== system carnot/Basic/Weather_and_Sun/Solar_Declination_Angle ==
  time : Inport
  S-Function : S-Function  FunctionName=solardeclination  SFunctionDeploymentMode=off  EnableBusSupport=off
  declination : Outport
  wires:
  time/1 -> S-Function/1
  S-Function/1 -> declination/1

== system carnot/Basic/Weather_and_Sun/Solar_Extraterrestrial_Radiation ==
  time : Inport
  S-Function : S-Function  FunctionName=solarextraterrestrialradiaton  SFunctionDeploymentMode=off  EnableBusSupport=off
  I_extra : Outport
  wires:
  S-Function/1 -> I_extra/1
  time/1 -> S-Function/1

== system carnot/Basic/Weather_and_Sun/Solar_Hour_Angle ==
  note: hourangle = (true_solar_time - 12*3600)*2*pi/24/3600
  time : Inport
  2*pi/(24*3600) : Gain  Gain=2*pi/(24*3600)
  Add : Sum  Inputs=+-
  Constant : Constant  Value=12*3600
  S-Function : S-Function  FunctionName=solartime  Parameters=timezone, longitude  SFunctionDeploymentMode=off  EnableBusSupport=off
  solar_hour_angle : Outport
  wires:
  time/1 -> S-Function/1
  S-Function/1 -> Add/1
  Add/1 -> 2*pi/(24*3600)/1
  2*pi/(24*3600)/1 -> solar_hour_angle/1
  Constant/1 -> Add/2

== system carnot/Basic/Weather_and_Sun/Solar_Position ==
  Solar_Position : S-Function  FunctionName=sunpos  Parameters=longi lati timezone  SFunctionDeploymentMode=off  EnableBusSupport=off
  Out1 : Outport
  wires:
  Solar_Position/1 -> Out1/1

== system carnot/Basic/Weather_and_Sun/Solar_Time ==
  time : Inport
  S-Function : S-Function  FunctionName=solartime  Parameters=timezone, longitude  SFunctionDeploymentMode=off  EnableBusSupport=off
  solartime : Outport
  wires:
  S-Function/1 -> solartime/1
  time/1 -> S-Function/1

== system carnot/Basic/Weather_and_Sun/WDB_Creator ==
  TimeValueComment : Inport
  Zenith_Angle : Inport  Port=2
  Azimuth_Angle : Inport  Port=3
  Solar_Radiation_beam_normal : Inport  Port=4
  Solar_Radiation_diffuse_horizontal : Inport  Port=5
  Temperature_Ambient : Inport  Port=6
  Temperature_Sky_Radiation : Inport  Port=7
  Relative_Humidity : Inport  Port=8
  Precipitation : Inport  Port=9
  Cloud_Index : Inport  Port=10
  Station_Pressure : Inport  Port=11
  Wind_Speed : Inport  Port=12
  Wind_Direction : Inport  Port=13
  Incidence_Angle_sun : Inport  Port=14
  Incidence_Angle_longitudinal : Inport  Port=15
  Incidence_Angle_transversal : Inport  Port=16
  Solar_Radiation_direct_surface : Inport  Port=17
  Solar_Radiation_diffuse_surface : Inport  Port=18
  Bus Creator : BusCreator  InitFcn=load WDB.mat  Inputs=18  OutDataTypeStr=Bus: WDB
  WDB : Outport
  wires:
  Bus Creator/1 -> WDB/1  "WDB"
  Solar_Radiation_diffuse_surface/1 -> Bus Creator/18  "Solar_Radiation_diffuse_surface"
  Solar_Radiation_direct_surface/1 -> Bus Creator/17  "Solar_Radiation_direct_surface"
  Incidence_Angle_transversal/1 -> Bus Creator/16  "Incidence_Angle_transversal"
  Incidence_Angle_longitudinal/1 -> Bus Creator/15  "Incidence_Angle_longitudinal"
  Incidence_Angle_sun/1 -> Bus Creator/14  "Incidence_Angle_sun"
  Wind_Direction/1 -> Bus Creator/13  "Wind_Direction"
  Wind_Speed/1 -> Bus Creator/12  "Wind_Speed"
  Station_Pressure/1 -> Bus Creator/11  "Station_Pressure"
  Cloud_Index/1 -> Bus Creator/10  "Cloud_Index"
  Precipitation/1 -> Bus Creator/9  "Precipitation"
  Relative_Humidity/1 -> Bus Creator/8  "Relative_Humidity"
  Temperature_Sky_Radiation/1 -> Bus Creator/7  "Temperature_Sky_Radiation"
  Temperature_Ambient/1 -> Bus Creator/6  "Temperature_Ambient"
  Solar_Radiation_diffuse_horizontal/1 -> Bus Creator/5  "Solar_Radiation_diffuse_horizontal"
  Azimuth_Angle/1 -> Bus Creator/3  "Azimuth_Angle"
  Zenith_Angle/1 -> Bus Creator/2  "Zenith_Angle"
  TimeValueComment/1 -> Bus Creator/1  "TimeValueComment"
  Solar_Radiation_beam_normal/1 -> Bus Creator/4  "Solar_Radiation_beam_normal"

== system carnot/Hydraulics/Flow_Diverter/increase_ID ==
  In1 : Inport
  Abs : Abs
  Bias : Bias  Bias=1
  Dot Product1 : DotProduct  InputSameDT=on  OutDataTypeStr=Inherit: Inherit via internal rule
  Sign : Signum
  Out1 : Outport
  wires:
  In1/1 -> Abs/1, Sign/1
  Dot Product1/1 -> Out1/1
  Abs/1 -> Bias/1
  Sign/1 -> Dot Product1/1
  Bias/1 -> Dot Product1/2

== system carnot/Hydraulics/Flow_Mixer/Calculate_fdiv ==
  ID_1 : Inport
  ID_2 : Inport  Port=2
  fdiv : Inport  Port=3
  Compare To Zero : simulink/Logic and Bit Operations/Compare To Zero  relop=<=  OutDataTypeStr=uint8
  Compare To Zero1 : simulink/Logic and Bit Operations/Compare To Zero  relop=<=  OutDataTypeStr=uint8
  Constant : Constant  Value=0
  Constant1 : Constant
  Gain1 : Gain  Gain=2
  Index Vector : MultiPortSwitch  DataPortOrder=Zero-based contiguous  zeroidx=on
  Memory : Memory
  MinMax2 : MinMax  Function=max  Inputs=2
  f_div : Outport
  wires:
  Index Vector/1 -> f_div/1
  Gain1/1 -> MinMax2/2
  Constant1/1 -> Index Vector/4
  fdiv/1 -> Memory/1
  Constant/1 -> Index Vector/3
  ID_2/1 -> Compare To Zero1/1
  ID_1/1 -> Compare To Zero/1
  MinMax2/1 -> Index Vector/1
  Compare To Zero/1 -> MinMax2/1
  Compare To Zero1/1 -> Gain1/1
  Memory/1 -> Index Vector/2

== system carnot/Hydraulics/Flow_Mixer_Thermostatic/Icontrol_fdiv ==
  ID_1 : Inport
  ID_2 : Inport  Port=2
  Twarm : Inport  Port=3
  Tset : Inport  Port=4
  Compare To Zero : simulink/Logic and Bit Operations/Compare To Zero  relop=<=  OutDataTypeStr=uint8
  Compare To Zero1 : simulink/Logic and Bit Operations/Compare To Zero  relop=<=  OutDataTypeStr=uint8
  Constant : Constant  Value=0
  Constant1 : Constant
  Gain : Gain  Gain=t1  SaturateOnIntegerOverflow=on  OutDataTypeStr=Inherit: Same as input  ParamDataTypeStr=Inherit: Same as input
  Gain1 : Gain  Gain=2
  Index Vector : MultiPortSwitch  DataPortOrder=Zero-based contiguous  zeroidx=on
  Integrator : Integrator  LimitOutput=on  UpperSaturationLimit=1  LowerSaturationLimit=0
  MinMax2 : MinMax  Function=max  Inputs=2
  diff_T : Sum  Inputs=-+  SaturateOnIntegerOverflow=on  InputSameDT=on  OutDataTypeStr=Inherit: Same as first input
  f_div : Outport
  wires:
  diff_T/1 -> Gain/1
  Gain/1 -> Integrator/1
  Twarm/1 -> diff_T/1
  Tset/1 -> diff_T/2
  Index Vector/1 -> f_div/1
  Gain1/1 -> MinMax2/2
  Constant1/1 -> Index Vector/4
  Integrator/1 -> Index Vector/2
  Constant/1 -> Index Vector/3
  ID_2/1 -> Compare To Zero1/1
  ID_1/1 -> Compare To Zero/1
  MinMax2/1 -> Index Vector/1
  Compare To Zero/1 -> MinMax2/1
  Compare To Zero1/1 -> Gain1/1

== system carnot/Hydraulics/Mixing_Valve/Calculate_fdiv ==
  ID_1 : Inport
  ID_2 : Inport  Port=2
  fdiv : Inport  Port=3
  Compare To Zero : simulink/Logic and Bit Operations/Compare To Zero  relop=<=  OutDataTypeStr=uint8
  Compare To Zero1 : simulink/Logic and Bit Operations/Compare To Zero  relop=<=  OutDataTypeStr=uint8
  Constant : Constant  Value=0
  Constant1 : Constant
  Gain1 : Gain  Gain=2
  Index Vector : MultiPortSwitch  DataPortOrder=Zero-based contiguous  zeroidx=on
  Memory : Memory
  MinMax2 : MinMax  Function=max  Inputs=2
  f_div : Outport
  wires:
  Index Vector/1 -> f_div/1
  Gain1/1 -> MinMax2/2
  Constant1/1 -> Index Vector/4
  fdiv/1 -> Memory/1
  Constant/1 -> Index Vector/3
  ID_2/1 -> Compare To Zero1/1
  ID_1/1 -> Compare To Zero/1
  MinMax2/1 -> Index Vector/1
  Compare To Zero/1 -> MinMax2/1
  Compare To Zero1/1 -> Gain1/1
  Memory/1 -> Index Vector/2

== system carnot/Hydraulics/Pump_Additional/select_clq ==
  THB : Inport
  Bus Selector : BusSelector  OutputSignals=DPConstant,DPLinear,DPQuadratic
  Mux2 : Mux  Inputs=3
  clq : Outport
  wires:
  Mux2/1 -> clq/1
  THB/1 -> Bus Selector/1
  Bus Selector/1 -> Mux2/1  "<DPConstant>"
  Bus Selector/2 -> Mux2/2  "<DPLinear>"
  Bus Selector/3 -> Mux2/3  "<DPQuadratic>"

== system carnot/Hydraulics/Valve/relFlowCoefficientFunction ==
  note: The definition of the flow coefficient Kv is:
      | Kv = Vdot * sqrt(1e5Pa/dp * density/1000kg/m³)
      | Vdot is the volumetric flow rate in m³/h
      | Kvs is the flow coefficient of the fully opened valve.
      | The relative flow coefficient psi is:
      | psi = Kv/Kvs
      |
      | Linear characteristics of the valve:
      | psi = psi_0 + m*h
      | with
      | h = H/H100 relative opening
      | psi_0 relative flow coeff. at h = 0
      | m inclination of the linear equation
      | psi should be 1 when h = 1, so: m = (1-psi_0)
      | psi = psi_0 + (1-psi_0)*h
      |
      | Equal percentage characteristics of the valve:
      | psi = psi_0 * e^(n*h)
      | with
      | n = ln(1/psi_0) inclination of the characteristics
      | the relative flow coefficient is:
      | psi = psi_0 * (1/psi_0)^h)
  h : Inport
  Constant : Constant  Value=vtyp
  EqualPercentageCharacteristic : Subsystem  TreatAsAtomicUnit=on  mask{psi_0=psi_0}
      mask prompts: psi_0 "Relative flow coefficient at zero opening"
      mask TypeOptions psi_0: psi_0/Value
  Index Vector : MultiPortSwitch
  LinearCharacteristic : Subsystem  TreatAsAtomicUnit=on  mask{psi_0=psi_0}
      mask prompts: psi_0 "Relative flow coefficient at zero opening"
      mask TypeOptions psi_0: psi_0/Value
  Switch Case : SwitchCase  CaseConditions={1,2}
  defaultLinear : Subsystem  TreatAsAtomicUnit=on  mask{psi_0=psi_0}
      mask prompts: psi_0 "Relative flow coefficient at zero opening"
      mask TypeOptions psi_0: psi_0/Value
  psi : Outport
  wires:
  defaultLinear/1(psi) -> Index Vector/4
  EqualPercentageCharacteristic/1(psi) -> Index Vector/3
  Switch Case/3 -> defaultLinear/Action
  Switch Case/2 -> EqualPercentageCharacteristic/Action
  LinearCharacteristic/1(psi) -> Index Vector/2
  h/1 -> LinearCharacteristic/1(h), EqualPercentageCharacteristic/1(h), defaultLinear/1(h)
  Switch Case/1 -> LinearCharacteristic/Action
  Constant/1 -> Switch Case/1, Index Vector/1
  Index Vector/1 -> psi/1  "relativeFlowCoeff"

== system carnot/Load/General/Data_from_File ==
  Constant : Constant
  FromWorkspace : FromWorkspace  VariableName=DataName  SampleTime=0  OutputAfterFinalValue=Holding final value
  Terminator : Terminator
  UnitDelay : UnitDelay  SampleTime=t_sample
  Data : Outport
  wires:
  FromWorkspace/1 -> Data/1  "Data"
  Constant/1 -> UnitDelay/1
  UnitDelay/1 -> Terminator/1

== system carnot/Load/General/Load_Data_Button ==

== system carnot/Load/General/Repeating_Profile ==
  Add : Sum  Inputs=1
  Pulse Generator : DiscretePulseGenerator  PulseType=Time based  Amplitude=rep_seq_y  Period=period  PulseWidth=rep_seq_d*100/period  PhaseDelay=rep_seq_t
  Out1 : Outport
  wires:
  Add/1 -> Out1/1
  Pulse Generator/1 -> Add/1

== system carnot/Load/Hot_Water_Tapping/DHW_Energy_Tapping ==
  Tc : Inport
  Rate Transition : RateTransition
  Rate Transition1 : RateTransition
  s_function : S-Function  FunctionName=dhw_EN13203  Parameters=times,energies,coeffs,dT_set,mdot_nom  SFunctionDeploymentMode=off  EnableBusSupport=off
  mdot : Outport
  Tset : Outport  Port=2
  wires:
  Rate Transition1/1 -> Tset/1
  Rate Transition/1 -> mdot/1
  Tc/1 -> s_function/1
  s_function/1 -> Rate Transition/1
  s_function/2 -> Rate Transition1/1

== system carnot/Load/Hot_Water_Tapping/EU_Tapping_Cycle ==
  Tc : Inport
  DHW_Energy_Tapping : $bdroot/Load/Hot_Water_Tapping/DHW_Energy_Tapping  mdot_nom=1  times=times  energies=energies  dT_set=dT_set  coeffs=mdot
  mdot : Outport
  Tset : Outport  Port=2
  wires:
  DHW_Energy_Tapping/1 -> mdot/1
  DHW_Energy_Tapping/2 -> Tset/1
  Tc/1 -> DHW_Energy_Tapping/1

== system carnot/Load/Hot_Water_Tapping/Hot_Water_Datafile ==
  THBcylinder : Inport
  Data_from_File : $bdroot/Load/General/Data_from_File  PathName=PathName  FileName=FileName  UserParam=off  DataName=DataName  t_sample=60
  T_cold_Water_Sine : $bdroot/Load/Hot_Water_Tapping/T_cold_Water_Sine  T=Tcold  Tamp=Tamp  dshift=dshift
  T_hot_water : Constant  Value=Thot
  Water_Tap : $bdroot/Load/Hot_Water_Tapping/Water_Tap  dia=0.02  p=2e5
  flow_diverter : $bdroot/Hydraulics/Flow_Diverter
  flow_mixer_thermostatic : $bdroot/Hydraulics/Flow_Mixer_Thermostatic  t=10
  mdot_DHWcalc : $bdroot/Load/Hot_Water_Tapping/mdot_DHWcalc  Commented=on  file=SFH_4P_200L_DHW  ext=.mat  dt=60
  THB_cylinder : Outport
  THB_tap : Outport  Port=2
  Tset : Outport  Port=3
  wires:
  Data_from_File/1 -> Water_Tap/1
  T_cold_Water_Sine/1 -> Water_Tap/2
  T_hot_water/1 -> Tset/1, flow_mixer_thermostatic/4
  Water_Tap/1 -> flow_diverter/1
  flow_mixer_thermostatic/2 -> flow_diverter/2
  flow_mixer_thermostatic/1 -> THB_tap/1
  THBcylinder/1 -> flow_mixer_thermostatic/1
  flow_diverter/1 -> THB_cylinder/1
  flow_diverter/2 -> flow_mixer_thermostatic/2
  flow_diverter/3 -> flow_mixer_thermostatic/3

== system carnot/Load/Hot_Water_Tapping/Hot_Water_EU_TappingCycle ==
  THBcylinder : Inport
  EU_Tapping_Cycle : $bdroot/Load/Hot_Water_Tapping/EU_Tapping_Cycle  eu_tap=L  dTbias=dTbias
  T_cold_water : Constant  Value=T_cold_water
  Water_Tap : $bdroot/Load/Hot_Water_Tapping/Water_Tap  dia=0.02  p=2e5
  flow_diverter : $bdroot/Hydraulics/Flow_Diverter
  flow_mixer_thermostatic : $bdroot/Hydraulics/Flow_Mixer_Thermostatic  t=1
  THB_cylinder : Outport
  THB_tap : Outport  Port=2
  Tset : Outport  Port=3
  wires:
  flow_mixer_thermostatic/1 -> THB_tap/1  "THBhot"
  EU_Tapping_Cycle/1 -> Water_Tap/1
  EU_Tapping_Cycle/2 -> flow_mixer_thermostatic/4, Tset/1  "Tset"
  T_cold_water/1 -> EU_Tapping_Cycle/1, Water_Tap/2
  flow_diverter/3 -> flow_mixer_thermostatic/3
  flow_diverter/2 -> flow_mixer_thermostatic/2
  flow_diverter/1 -> THB_cylinder/1  "THBcold"
  THBcylinder/1 -> flow_mixer_thermostatic/1
  flow_mixer_thermostatic/2 -> flow_diverter/2
  Water_Tap/1 -> flow_diverter/1

== system carnot/Load/Hot_Water_Tapping/Hot_Water_Energy_Profile ==
  THBcylinder : Inport
  DHW_Energy_Tapping : $bdroot/Load/Hot_Water_Tapping/DHW_Energy_Tapping  mdot_nom=mdot_nom  times=times  energies=energies  dT_set=dT_set  coeffs=coeffs
  T_cold_water_const : Constant  Value=Tcw
  Water_Tap : $bdroot/Load/Hot_Water_Tapping/Water_Tap  dia=0.02  p=2e5
  flow_diverter : $bdroot/Hydraulics/Flow_Diverter
  flow_mixer_thermostatic : $bdroot/Hydraulics/Flow_Mixer_Thermostatic  t=10
  THB_cylinder : Outport
  THB_tap : Outport  Port=2
  Tset : Outport  Port=3
  wires:
  DHW_Energy_Tapping/2 -> Tset/1, flow_mixer_thermostatic/4
  DHW_Energy_Tapping/1 -> Water_Tap/1
  T_cold_water_const/1 -> Water_Tap/2, DHW_Energy_Tapping/1
  Water_Tap/1 -> flow_diverter/1
  flow_mixer_thermostatic/2 -> flow_diverter/2
  flow_mixer_thermostatic/1 -> THB_tap/1
  THBcylinder/1 -> flow_mixer_thermostatic/1
  flow_diverter/1 -> THB_cylinder/1
  flow_diverter/2 -> flow_mixer_thermostatic/2
  flow_diverter/3 -> flow_mixer_thermostatic/3

== system carnot/Load/Hot_Water_Tapping/Hot_Water_T_Mdot_Profile ==
  THBcylinder : Inport
  T_cold_Water_Sine : $bdroot/Load/Hot_Water_Tapping/T_cold_Water_Sine  T=Tcold  Tamp=Tamp  dshift=dshift
  T_hot_water : Constant  Value=Thot
  Water_Tap : $bdroot/Load/Hot_Water_Tapping/Water_Tap  dia=0.02  p=2e5
  flow_diverter : $bdroot/Hydraulics/Flow_Diverter
  flow_mixer_thermostatic : $bdroot/Hydraulics/Flow_Mixer_Thermostatic  t=10
  mdot_rep_seq : $bdroot/Load/Hot_Water_Tapping/mdot_rep_seq  period=period  rep_seq_t=rep_seq_t  rep_seq_d=rep_seq_d  rep_seq_y=rep_seq_y
  THB_cylinder : Outport
  THB_tap : Outport  Port=2
  Tset : Outport  Port=3
  wires:
  flow_diverter/3 -> flow_mixer_thermostatic/3
  flow_diverter/2 -> flow_mixer_thermostatic/2
  flow_diverter/1 -> THB_cylinder/1
  THBcylinder/1 -> flow_mixer_thermostatic/1
  flow_mixer_thermostatic/1 -> THB_tap/1
  flow_mixer_thermostatic/2 -> flow_diverter/2
  Water_Tap/1 -> flow_diverter/1
  T_hot_water/1 -> flow_mixer_thermostatic/4, Tset/1
  T_cold_Water_Sine/1 -> Water_Tap/2
  mdot_rep_seq/1 -> Water_Tap/1

== system carnot/Load/Hot_Water_Tapping/T_cold_Water_Location ==
  Sine Wave : Sin  Amplitude=Tamp  Bias=T  Frequency=(2*pi/365/24/3600)  Phase=(2*pi*dshift/365)  SampleTime=0
  Tc : Outport  InitialOutput=0
  wires:
  Sine Wave/1 -> Tc/1

== system carnot/Load/Hot_Water_Tapping/T_cold_Water_Season ==
  S-Function : S-Function  FunctionName=season_temperature  Parameters=month1 temp1 month2 temp2 form  SFunctionDeploymentMode=off  EnableBusSupport=off
  Tc : Outport
  wires:
  S-Function/1 -> Tc/1

== system carnot/Load/Hot_Water_Tapping/T_cold_Water_Sine ==
  Sine Wave : Sin  Amplitude=Tamp  Bias=T  Frequency=(2*pi/365/24/3600)  Phase=(2*pi*dshift/365)  SampleTime=0
  Tc : Outport  InitialOutput=0
  wires:
  Sine Wave/1 -> Tc/1

== system carnot/Load/Hot_Water_Tapping/Water_Tap ==
  mdot : Inport
  Tc : Inport  Port=2
  basic_create_THB : $bdroot/Basic/Hydraulics/basic_create_THB  p=p  fluid=Water  mix=mix  mix2=0  mix3=0  dia=dia  hgt=0  mID=No Pressure Drop
  THB : Outport
  wires:
  mdot/1 -> basic_create_THB/1
  Tc/1 -> basic_create_THB/2
  basic_create_THB/1 -> THB/1
